simulink model "controladorLQG_Discreto_sim"  (R2020a)
settings: Solver=VariableStepAuto  StartTime=0.0  StopTime=20  FixedStep=-1  RelTol=1e-3
values from neighbouring files (symbols this model uses):
  A = [  sigma      tau    -r*sigma ... (first row only)    [controlador_LQR.m]
  Ad = sysd.a    [controlador_LQR.m]
  B = [alfa; 0; beta]    [controlador_LQR.m]
  Bd = sysd.b    [controlador_LQR.m]
  C = [0 1 0]    [controlador_LQR.m]
  D = zeros(size(C,1),size(B,2))    [controlador_LQR.m]
  L = 0.0752    [controlador_LQR.m]
  sigma = (2*(Rm*b - Ke*Km)*(Jb + Mb*L^2 + Mb*L*r))/den    [controlador_LQR.m]
  sysKFd = ss(Ad-Ld*C,[Bd Ld],eye(3),0*[Bd Ld])    [controlador_LQR.m]
undefined symbols (not defined in the file or in its folder): Discrete, K, kalmf, Klqr, Krd, Llqe, Time
libraries: simulink x6, ctrlSharedLib x1
settings Model: Creator=Matheus  LastModifiedBy=mathe
settings DataIOCC: ReturnWorkspaceOutputs=off
settings DebuggingCC: ArithmeticOperatorsInVariantConditions=warning
settings SFSimCC: SimUseLocalCustomCode=off  CustomCodeUndefinedFunction=UseInterfaceOnly
settings RTWCC: RTWUseLocalCustomCode=off
settings CodeAppCC: StateflowObjectComments=on

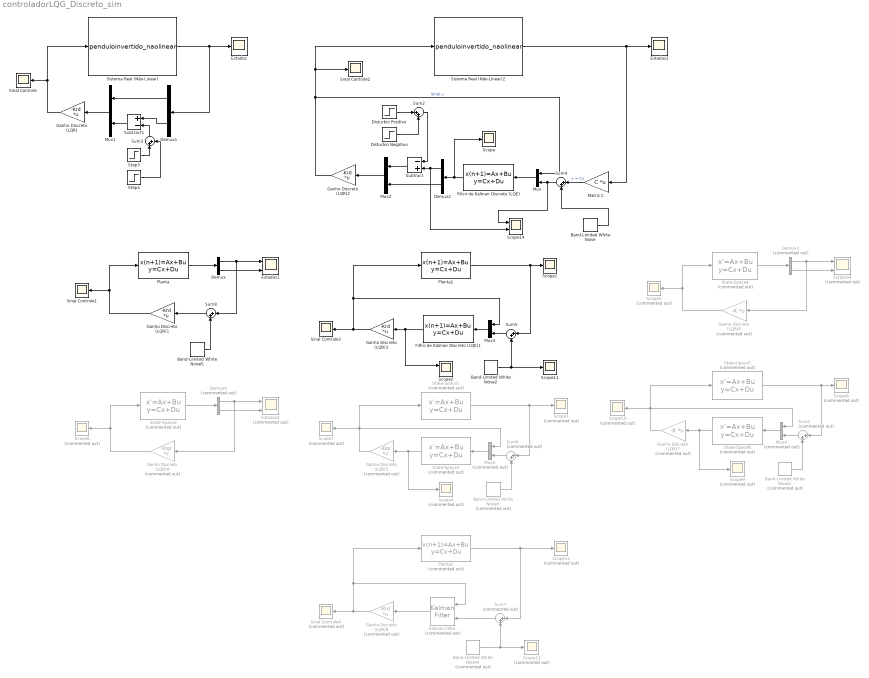
== system controladorLQG_Discreto_sim ==
  Band-Limited White Noise : simulink/Sources/Band-Limited White Noise  Cov=0.0001  Ts=0.05  seed=[23341]
  Band-Limited White Noise1 : simulink/Sources/Band-Limited White Noise  Commented=on  Cov=0.000001  Ts=0.1  seed=[23341]
  Band-Limited White Noise2 : simulink/Sources/Band-Limited White Noise  Cov=.0001  Ts=0.05  seed=[23341]
  Band-Limited White Noise3 : simulink/Sources/Band-Limited White Noise  Commented=on  Cov=0.1  Ts=0.1  seed=[23341]
  Band-Limited White Noise4 : simulink/Sources/Band-Limited White Noise  Commented=on  Cov=0  Ts=0.05  seed=[23341]
  Band-Limited White Noise5 : simulink/Sources/Band-Limited White Noise  Cov=.001  Ts=0.05  seed=[23341]
  Demux : Demux  Outputs=2
  Demux1 : Demux  Outputs=2
  Demux2 : Demux  Outputs=2
  Demux3 : Demux  Commented=on  Outputs=2
  Demux4 : Demux  Commented=on  Outputs=2
  Disturbio Negativo : Step  Time=10.5  After=-3.14/20
  Disturbio Positivo : Step  Time=10  After=3.14/20
  Estados : Scope
  Estados1 : Scope  NumInputPorts=2
  Estados2 : Scope
  Estados3 : Scope  Commented=on  NumInputPorts=2
  Estados4 : Scope  Commented=on  NumInputPorts=2
  Filtro de Kalman Discreto (LQE) : DiscreteStateSpace  A=sysKFd.a  B=sysKFd.b  C=sysKFd.c  D=sysKFd.d  InitialCondition=[0 0]  SampleTime=-1
  Filtro de Kalman Discreto (LQE)1 : DiscreteStateSpace  A=sysKFd.a  B=sysKFd.b  C=sysKFd.c  D=sysKFd.d  InitialCondition=[0 0]  SampleTime=0.05
  Ganho Discreto (LQR){,1..3} (4 alike) : Gain  Gain=-Krd  Multiplication=Matrix(K*u) (u vector)
  Ganho Discreto (LQR)4 : Gain  Commented=on  Gain=-Klqr  Multiplication=Matrix(K*u) (u vector)
  Ganho Discreto (LQR)5 : Gain  Commented=on  Gain=-Klqr  Multiplication=Matrix(K*u) (u vector)
  Ganho Discreto (LQR)6 : Gain  Commented=on  Gain=-K  Multiplication=Matrix(K*u) (u vector)
  Ganho Discreto (LQR)7 : Gain  Commented=on  Gain=-K  Multiplication=Matrix(K*u) (u vector)
  Ganho Discreto (LQR)8 : Gain  Commented=on  Gain=-Krd  Multiplication=Matrix(K*u) (u vector)
  Kalman Filter : ctrlSharedLib/Kalman Filter  Commented=on  TimeDomain=Discrete-Time  UseCurrentEstimator=on  ModelSource=Individual A, B, C, D matrices  ModelSourceVariable=ss(0.95,1,1,0,1)  A=kalmf.a  B=kalmf.b  C=kalmf.c  D=kalmf.d  NumberOfStates=1  NumberOfInputs=1  NumberOfOutputs=1  InitialEstimateSource=Dialog  X0=0  P0=10  UseK=off  UseGH=off  NumberOfProcessNoiseInputs=1  G=1  TimeInvariantG=on  H=0  TimeInvariantH=on  Q=1  TimeInvariantQ=on  R=1  TimeInvariantR=on  N=0  TimeInvariantN=on  AddInputPort=on  AddEnablePort=off  OutputEstimatedY=off  OutputP=off  Ts=0.05
  Matriz C : Gain  Gain=C  Multiplication=Matrix(K*u) (u vector)
  Mux{,1..3} (4 alike) : Mux  Inputs=2
  Mux4 : Mux  Commented=on  Inputs=2
  Mux5 : Mux  Commented=on  Inputs=2
  Planta : DiscreteStateSpace  A=Ad  B=Bd  C=[eye(2); C]  D=[D; 0; 0]  InitialCondition=[pi/3 0]  SampleTime=0.05
  Planta1 : DiscreteStateSpace  A=Ad  B=Bd  C=C  D=D  InitialCondition=[pi/6 0]  SampleTime=0.05
  Planta2 : DiscreteStateSpace  Commented=on  A=Ad  B=Bd  C=C  D=D  InitialCondition=[0.10 -0.10]  SampleTime=0.05
  Scope : Scope
  Scope1 : Scope
  Scope{3..10,12..13} (10 alike) : Scope  Commented=on
  Scope11 : Scope
  Scope14 : Scope  NumInputPorts=2
  Scope2 : Scope  NumInputPorts=2
  Sinal Controle{,1..3} (4 alike) : Scope
  Sinal Controle4 : Scope  Commented=on
  Sistema Real (Não-Linear) : S-Function  InitFcn=try, set_param(gcb,'FunctionName','penduloinvertido_naolinear'), end  FunctionName=penduloinvertido_naolinear  SFunctionModules=penduloinvertido_naolinear_wrapper  SFunctionDeploymentMode=off  EnableBusSupport=off  mask(S-Function Builder){}
      mask help: Simulink:masks:SFunctionBuilder_MD
      mask init:
      | val = [[.9  0.75 0.75 1 1 .9 .9 1]',[1 1 0.75 0.75 .9 .9 1 .9]'];try , sys = get_param(gcb,'SfunBuilderFcnName');if isempty(sys), sys = get_param(gcb,'FunctionName'); end,catch, sys = get_param(gcb,'FunctionName'); end
      settings: CopyFcn=set_param(gcbh,'LinkStatus','none')  PreSaveFcn=try, set_param(gcb,'FunctionName','penduloinvertido_naolinear'), end  OpenFcn=sfunctionwizard(gcbh)
      mask Display: plot(val(:,1),val(:,2)),disp(sys), port_label('input',1,'u0'), port_label('output',1,'y0')
  Sistema Real (Não-Linear)2 : S-Function  InitFcn=try, set_param(gcb,'FunctionName','penduloinvertido_naolinear'), end  FunctionName=penduloinvertido_naolinear  SFunctionModules=penduloinvertido_naolinear_wrapper  SFunctionDeploymentMode=off  EnableBusSupport=off  mask(S-Function Builder){}
      mask help: Simulink:masks:SFunctionBuilder_MD
      mask init: same as controladorLQG_Discreto_sim/Sistema Real (Não-Linear)
      settings: CopyFcn=set_param(gcbh,'LinkStatus','none')  PreSaveFcn=try, set_param(gcb,'FunctionName','penduloinvertido_naolinear'), end  OpenFcn=sfunctionwizard(gcbh)
      mask Display: plot(val(:,1),val(:,2)),disp(sys), port_label('input',1,'u0'), port_label('output',1,'y0')
  State-Space1 : StateSpace  Commented=on  A=A  B=B  C=C  D=D  InitialCondition=[0.1/sigma 0]
  State-Space2 : StateSpace  Commented=on  A=A  B=B  C=[eye(2); C]  D=[D; 0; 0]  InitialCondition=[0.1 0]
  State-Space3 : StateSpace  Commented=on  A=A-Llqe*C  B=[B Llqe]  C=eye(2)  D=zeros(2,2)  InitialCondition=0
  State-Space4 : StateSpace  Commented=on  A=A  B=B  C=[eye(2); C]  D=[D; 0; 0]  InitialCondition=[0.10 0]
  State-Space5 : StateSpace  Commented=on  A=A  B=B  C=C  D=D  InitialCondition=[0.25 0.1]
  State-Space6 : StateSpace  Commented=on  A=A-L*C  B=[B L]  C=eye(2)  D=zeros(2,2)  InitialCondition=[0.25 0.1]
  Step3 : Step  Time=10  After=0
  Step4 : Step  Time=10.5  After=0
  Subtract : Sum  Inputs=-+
  Subtract1 : Sum  Inputs=+-
  Sum1 : Sum  Commented=on  Inputs=|++
  Sum{2..5,8} (5 alike) : Sum  Inputs=|++
  Sum6 : Sum  Commented=on  Inputs=|++
  Sum7 : Sum  Commented=on  Inputs=|++
  wires:
  Sistema Real (Não-Linear)2/1 -> Estados2/1, Matriz C/1
  Ganho Discreto (LQR)2/1 -> Sistema Real (Não-Linear)2/1, Sinal Controle2/1, Mux/1  "Sinal u"
  Filtro de Kalman Discreto (LQE)/1 -> Scope/1, Demux2/1
  Mux/1 -> Filtro de Kalman Discreto (LQE)/1
  Disturbio Positivo/1 -> Sum2/1
  Disturbio Negativo/1 -> Sum2/2
  Ganho Discreto (LQR)/1 -> Sistema Real (Não-Linear)/1, Sinal Controle/1
  Step3/1 -> Sum3/1
  Demux1/2 -> Subtract1/1
  Step4/1 -> Sum3/2
  Demux1/1 -> Mux1/1
  Sum3/1 -> Subtract1/2
  Mux1/1 -> Ganho Discreto (LQR)/1
  Subtract1/1 -> Mux1/2
  Sistema Real (Não-Linear)/1 -> Demux1/1, Estados/1
  Mux2/1 -> Ganho Discreto (LQR)2/1
  Sum4/1 -> Scope14/1, Mux/2
  Matriz C/1 -> Sum4/1  "y = Cx"
  Band-Limited White Noise/1 -> Sum4/2
  Planta/1 -> Demux/1
  Demux/1 -> Sum8/1, Estados1/1
  Ganho Discreto (LQR)1/1 -> Planta/1, Sinal Controle1/1
  Mux3/1 -> Filtro de Kalman Discreto (LQE)1/1
  Planta1/1 -> Sum5/1, Scope1/1
  Sum5/1 -> Mux3/2
  Demux/2 -> Estados1/2
  Ganho Discreto (LQR)4/1 -> State-Space2/1, Scope8/1
  State-Space3/1 -> Scope4/1, Ganho Discreto (LQR)5/1
  State-Space1/1 -> Scope3/1, Sum6/1
  Mux5/1 -> State-Space3/1
  Ganho Discreto (LQR)5/1 -> Scope7/1, State-Space1/1, Mux5/1
  Sum6/1 -> Mux5/2
  Band-Limited White Noise3/1 -> Sum6/2
  State-Space2/1 -> Demux4/1
  Demux4/1 -> Estados3/1, Ganho Discreto (LQR)4/1
  Demux4/2 -> Estados3/2
  Band-Limited White Noise2/1 -> Scope11/1, Sum5/2
  Filtro de Kalman Discreto (LQE)1/1 -> Scope2/1, Ganho Discreto (LQR)3/1
  Ganho Discreto (LQR)6/1 -> State-Space4/1, Scope5/1
  Demux3/2 -> Estados4/2
  State-Space4/1 -> Demux3/1
  Demux3/1 -> Estados4/1, Ganho Discreto (LQR)6/1
  Ganho Discreto (LQR)7/1 -> Scope10/1, State-Space5/1, Mux4/1
  State-Space5/1 -> Scope6/1, Sum1/1
  Mux4/1 -> State-Space6/1
  Sum1/1 -> Mux4/2
  State-Space6/1 -> Scope9/1, Ganho Discreto (LQR)7/1
  Band-Limited White Noise1/1 -> Sum1/2
  Ganho Discreto (LQR)8/1 -> Kalman Filter/1, Planta2/1, Sinal Controle4/1
  Kalman Filter/1 -> Ganho Discreto (LQR)8/1
  Band-Limited White Noise4/1 -> Sum7/2, Scope13/1
  Sum7/1 -> Kalman Filter/2
  Planta2/1 -> Sum7/1, Scope12/1
  Ganho Discreto (LQR)3/1 -> Planta1/1, Mux3/1, Sinal Controle3/1
  Sum8/1 -> Ganho Discreto (LQR)1/1
  Band-Limited White Noise5/1 -> Sum8/2
  Subtract/1 -> Mux2/1
  Demux2/2 -> Mux2/2
  Demux2/1 -> Scope14/2, Subtract/2
  Sum2/1 -> Subtract/1
